simulink model "mecanum_sim"  (R2019b)
settings: Solver=VariableStepAuto  StartTime=0.0  StopTime=inf  RelTol=1e-3
InitFcn:
  | mecanum_init
values from neighbouring files (symbols this model uses):
  J = (1/r)*[1 1 a+b ... (first row only)    [mecanum_init.m]
undefined symbols (not defined in the file or in its folder): J3
libraries: aerolibutil x1, aerolibanimutils x1
settings Model: Creator=giull  LastModifiedBy=giull

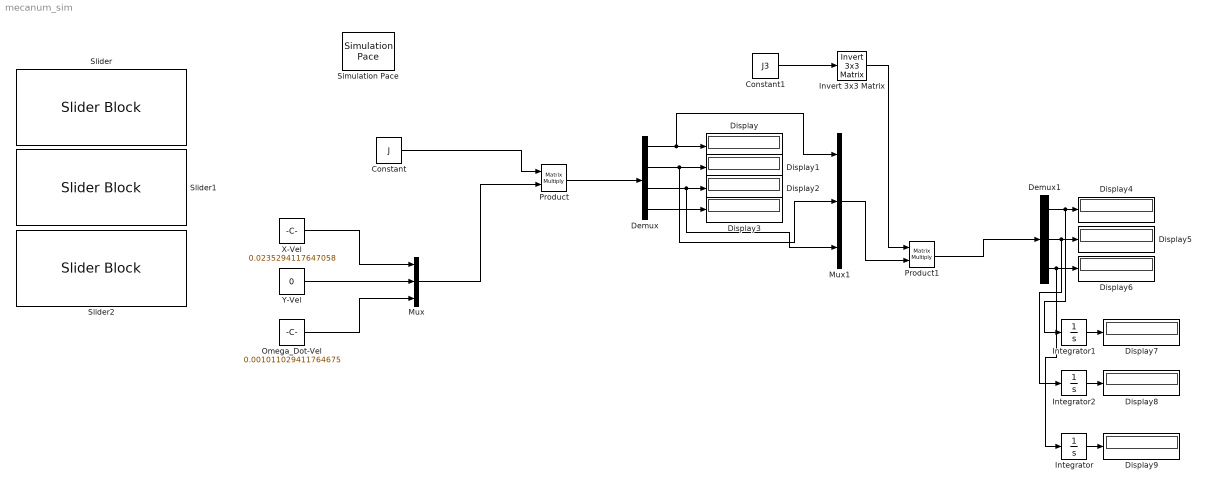
== system mecanum_sim ==
  Constant : Constant  Value=J
  Constant1 : Constant  Value=J3
  Demux : Demux
  Demux1 : Demux  Outputs=3
  Display{,1..9} (10 alike) : Display
  Integrator : Integrator
  Integrator1 : Integrator
  Integrator2 : Integrator
  Invert 3x3 Matrix : aerolibutil/Invert  3x3 Matrix
  Mux : Mux  Inputs=3
  Mux1 : Mux  Inputs=3
  Omega_Dot-Vel : Constant  Value=0.001011029411764675
  Product : Product  Multiplication=Matrix(*)
  Product1 : Product  Multiplication=Matrix(*)
  Simulation Pace : aerolibanimutils/Simulation Pace  SimulationPace=1  SleepMode=Auto  OutputPaceError=off  SampleTime=1/30
  Slider : SliderBlock  ScaleMin=-2  ScaleMax=2
  Slider1 : SliderBlock  ScaleMin=-2  ScaleMax=2
  Slider2 : SliderBlock  ScaleMin=-0.5  ScaleMax=0.5
  X-Vel : Constant  Value=0.0235294117647058
  Y-Vel : Constant  Value=0
  wires:
  Constant/1 -> Product/1
  Y-Vel/1 -> Mux/2
  X-Vel/1 -> Mux/1
  Omega_Dot-Vel/1 -> Mux/3
  Product/1 -> Demux/1
  Mux/1 -> Product/2
  Demux/2 -> Mux1/2, Display1/1
  Demux/1 -> Mux1/1, Display/1
  Demux/3 -> Mux1/3, Display2/1
  Demux/4 -> Display3/1
  Constant1/1 -> Invert 3x3 Matrix/1
  Product1/1 -> Demux1/1
  Demux1/1 -> Integrator1/1, Display4/1
  Demux1/2 -> Integrator2/1, Display5/1
  Demux1/3 -> Integrator/1, Display6/1
  Invert 3x3 Matrix/1 -> Product1/1
  Mux1/1 -> Product1/2
  Integrator/1 -> Display9/1
  Integrator2/1 -> Display8/1
  Integrator1/1 -> Display7/1
